simulink library "communications_lib"  (Simulink 8.1)
settings: Solver=ode45  StartTime=0.0  StopTime=10.0  RelTol=1e-3
values from neighbouring files (symbols this model uses):
  Ts = 100E-6    (= 0.0001)    [BANSHEE_init.m]
undefined symbols (not defined in the file or in its folder): DMS_slave_lib, DMSCommands
libraries: goose_lib x5, udp_powerfactor_lib x3, LoadProfiles_lib x1, NREL_UDP_lib x1, rtlab x1
settings Model: Creator=re25624  LastModifiedBy=pkoralew

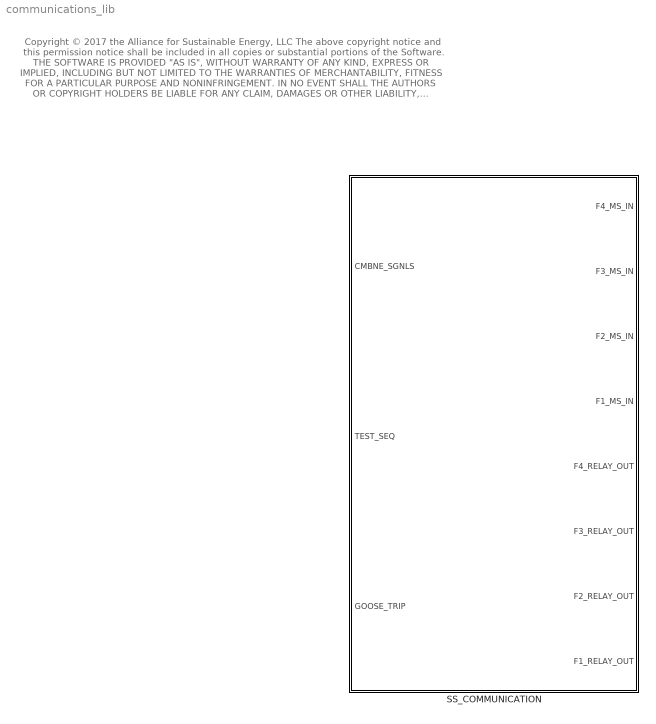
== system communications_lib ==
  note: Copyright © 2017 the Alliance for Sustainable Energy, LLC
      |
      | The above copyright notice and this permission notice shall be included in all copies or substantial portions of the Software.
      |
      | THE SOFTWARE IS PROVIDED "AS IS", WITHOUT WARRANTY OF ANY KIND, EXPRESS OR IMPLIED, INCLUDING
      | BUT NOT LIMITED TO THE WARRANTIES OF MERCHANTABILITY, FITNESS FOR A PARTICULAR PURPOSE AND
      | NONINFRINGEMENT. IN NO EVENT SHALL THE AUTHORS OR COPYRIGHT HOLDERS BE LIABLE FOR ANY CLAIM,
      |  DAMAGES OR OTHER LIABILITY, WHETHER IN AN ACTION OF CONTRACT, TORT OR OTHERWISE, ARISING FROM,
      | OUT OF OR IN CONNECTION WITH THE SOFTWARE OR THE USE OR OTHER DEALINGS IN THE SOFTWARE
  SS_COMMUNICATION : Subsystem

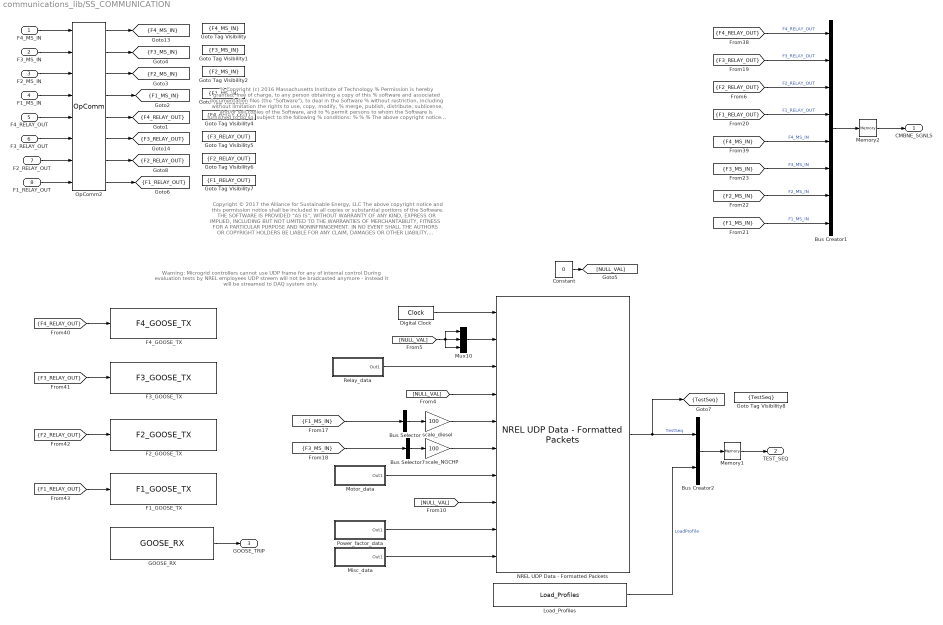
== system communications_lib/SS_COMMUNICATION ==
  note: Copyright © 2017 the Alliance for Sustainable Energy, LLC
      |
      | The above copyright notice and this permission notice shall be included in all copies or substantial portions of the Software.
      |
      | THE SOFTWARE IS PROVIDED "AS IS", WITHOUT WARRANTY OF ANY KIND, EXPRESS OR IMPLIED, INCLUDING
      | BUT NOT LIMITED TO THE WARRANTIES OF MERCHANTABILITY, FITNESS FOR A PARTICULAR PURPOSE AND
      | NONINFRINGEMENT. IN NO EVENT SHALL THE AUTHORS OR COPYRIGHT HOLDERS BE LIABLE FOR ANY CLAIM,
      |  DAMAGES OR OTHER LIABILITY, WHETHER IN AN ACTION OF CONTRACT, TORT OR OTHERWISE, ARISING FROM,
      | OUT OF OR IN CONNECTION WITH THE SOFTWARE OR THE USE OR OTHER DEALINGS IN THE SOFTWARE
  note: % Copyright (c) 2016 Massachusetts Institute of Technology
      | % Permission is hereby granted, free of charge, to any person obtaining a copy of this
      | % software and associated documentation files (the "Software"), to deal in the Software
      | % without restriction, including without limitation the rights to use, copy, modify,
      | % merge, publish, distribute, sublicense, and/or sell copies of the Software, and to
      | % permit persons to whom the Software is furnished to do so, subject to the following
      | % conditions:
      | %
      | %
      | % The above copyright notice and this permission notice shall be included in
      | % all copies or substantial portions of the Software.
      | %
      | % THE SOFTWARE IS PROVIDED "AS IS", WITHOUT WARRANTY OF ANY KIND, EXPRESS OR IMPLIED,
      | % INCLUDING BUT NOT LIMITED TO THE WARRANTIES OF MERCHANTABILITY, FITNESS FOR A
      | % PARTICULAR PURPOSE AND NONINFRINGEMENT. IN NO EVENT SHALL THE AUTHORS OR COPYRIGHT
      | % HOLDERS BE LIABLE FOR ANY CLAIM, DAMAGES OR OTHER LIABILITY, WHETHER IN AN ACTION
      | % OF CONTRACT, TORT OR OTHERWISE, ARISING FROM, OUT OF OR IN CONNECTION WITH THE
      | % SOFTWARE OR THE USE OR OTHER DEALINGS IN THE SOFTWARE.
      | %
      | %
      | %%
  note: Warning: Microgrid controllers cannot use UDP frame for any of internal control
      | During evaluation tests by NREL employees UDP streem will not be bradcasted anymore - instead it will
      | be streamed to DAQ system only.
  F4_MS_IN : Inport
  F3_MS_IN : Inport  Port=2
  F2_MS_IN : Inport  Port=3
  F1_MS_IN : Inport  Port=4
  F4_RELAY_OUT : Inport  Port=5
  F3_RELAY_OUT : Inport  Port=6
  F2_RELAY_OUT : Inport  Port=7
  F1_RELAY_OUT : Inport  Port=8
  Bus Creator1 : BusCreator  Inputs=8
  Bus Creator2 : BusCreator  Inputs=2
  Bus Selector : BusSelector  OutputSignals=DIESEL_DATA.gen.gal_per_hr,DIESEL_DATA.cb.relay_out.m.Vpu  OutputAsBus=on
  Bus Selector7 : BusSelector  OutputSignals=NG_CHP_DATA.cb.relay_out.m.Vpu,NG_CHP_DATA.CHPData.TempActual,NG_CHP_DATA.CHPData.Thermal data.Heat Recovered; MBtu/hr,NG_CHP_DATA.CHPData.Thermal data.Nm^3 per hour NG fuel usage,NG_CHP_DATA.CHPData.Thermal data.CO2 lbm/hr,NG_CHP_DATA.CHPData.HeatFromBoiler MBtu/hr,NG_CHP_DATA.CHPData.CHPHeatContribution MBtu/hr,NG_CHP_DATA.CHPData.Boiler_Nm^3/hr ,NG_CHP_DATA.CHPData.Boiler lbm/hr CO2  OutputAsBus=on
  Constant : Constant  Value=0
  Digital Clock : DigitalClock  SampleTime=Ts
  F1_GOOSE_TX : goose_lib/F1_GOOSE_TX
  F2_GOOSE_TX : goose_lib/F2_GOOSE_TX
  F3_GOOSE_TX : goose_lib/F3_GOOSE_TX
  F4_GOOSE_TX : goose_lib/F4_GOOSE_TX
  "GOOSE_RX " : goose_lib/GOOSE_RX 
  Goto Tag Visibility : GotoTagVisibility  GotoTag=F4_MS_IN
  Goto Tag Visibility1 : GotoTagVisibility  GotoTag=F3_MS_IN
  Goto Tag Visibility2 : GotoTagVisibility  GotoTag=F2_MS_IN
  Goto Tag Visibility3 : GotoTagVisibility  GotoTag=F1_MS_IN
  Goto Tag Visibility4 : GotoTagVisibility  GotoTag=F4_RELAY_OUT
  Goto Tag Visibility5 : GotoTagVisibility  GotoTag=F3_RELAY_OUT
  Goto Tag Visibility6 : GotoTagVisibility  GotoTag=F2_RELAY_OUT
  Goto Tag Visibility7 : GotoTagVisibility  GotoTag=F1_RELAY_OUT
  Goto Tag Visibility8 : GotoTagVisibility  GotoTag=TestSeq
  Load_Profiles : LoadProfiles_lib/Load_Profiles
  Memory1 : Memory
  Memory2 : Memory
  Misc_data : Subsystem
  Motor_data : Subsystem
  Mux10 : Mux  Inputs=3
  NREL UDP Data - Formatted Packets : NREL_UDP_lib/NREL UDP Data - Formatted Packets  ProfileID=2  NumOfWaveforms=[3, 1, 1]  NumOfRelays=[59, [1, 1, 1000, 100]]  NumOfBatteries=0  NumOfDieselGensets=[1, [100, 100]]  NumOfNGCHPGensets=[1, [100, 100, 100, 100, 100, 100, 100, 100, 100]]  NumOfMotors=2  NumOfPVs=0  NumOfPF=[3, 1000]  NumOfMiscellaneousDataScales=2  NumOfMiscellaneousDataSignalsScales=[[50, 1], [8, 1]]
  OpComm2 : rtlab/OpComm  nbport=8  groupe_acq=1  subsys_rate=0  st=0  Synchronization=on  Interpolation=on  Threshold=1.0  Missed_Data=off  Sim_Time=off  Samples=off  dynSigOut=off  from_console=0  warning_done=off  writeOpCommFile=off  Offset=off
  Power_factor_data : Subsystem
  Relay_data : Subsystem
  scale_NGCHP : Gain  Gain=100
  scale_diesel : Gain  Gain=100
  CMBNE_SGNLS : Outport
  TEST_SEQ : Outport  Port=2
  GOOSE_TRIP : Outport  Port=3
  tag scope: F1_MS_IN=scoped, F1_RELAY_OUT=scoped, F2_MS_IN=scoped, F2_RELAY_OUT=scoped, F3_MS_IN=scoped, F3_RELAY_OUT=scoped, F4_MS_IN=scoped, F4_RELAY_OUT=scoped, TestSeq=scoped
  wires:
  Bus Creator2/1 -> Memory1/1
  NREL UDP Data - Formatted Packets/1 -> Bus Creator2/1, [TestSeq]  "TestSeq"
  Motor_data/1(Out1) -> NREL UDP Data - Formatted Packets/7
  Misc_data/1(Out1) -> NREL UDP Data - Formatted Packets/10
  Relay_data/1(Out1) -> NREL UDP Data - Formatted Packets/3
  "GOOSE_RX "/1 -> GOOSE_TRIP/1
  [F1_RELAY_OUT] -> F1_GOOSE_TX/1
  [F2_RELAY_OUT] -> F2_GOOSE_TX/1
  [F3_RELAY_OUT] -> F3_GOOSE_TX/1
  [F4_RELAY_OUT] -> F4_GOOSE_TX/1
  [F4_MS_IN] -> Bus Creator1/5  "F4_MS_IN"
  [F4_RELAY_OUT] -> Bus Creator1/1  "F4_RELAY_OUT"
  OpComm2/8 -> [F1_RELAY_OUT]
  OpComm2/7 -> [F2_RELAY_OUT]
  OpComm2/6 -> [F3_RELAY_OUT]
  OpComm2/5 -> [F4_RELAY_OUT]
  OpComm2/4 -> [F1_MS_IN]
  OpComm2/3 -> [F2_MS_IN]
  OpComm2/2 -> [F3_MS_IN]
  OpComm2/1 -> [F4_MS_IN]
  F3_RELAY_OUT/1 -> OpComm2/6
  F4_RELAY_OUT/1 -> OpComm2/5
  F4_MS_IN/1 -> OpComm2/1
  Digital Clock/1 -> NREL UDP Data - Formatted Packets/1
  [F2_MS_IN] -> Bus Creator1/7  "F2_MS_IN"
  [F3_MS_IN] -> Bus Creator1/6  "F3_MS_IN"
  [F3_RELAY_OUT] -> Bus Creator1/2  "F3_RELAY_OUT"
  [F1_RELAY_OUT] -> Bus Creator1/4  "F1_RELAY_OUT"
  [F2_RELAY_OUT] -> Bus Creator1/3  "F2_RELAY_OUT"
  [F1_MS_IN] -> Bus Creator1/8  "F1_MS_IN"
  Bus Creator1/1 -> Memory2/1
  Memory2/1 -> CMBNE_SGNLS/1
  scale_NGCHP/1 -> NREL UDP Data - Formatted Packets/6
  Bus Selector7/1 -> scale_NGCHP/1
  scale_diesel/1 -> NREL UDP Data - Formatted Packets/5
  [F3_MS_IN] -> Bus Selector7/1
  Bus Selector/1 -> scale_diesel/1
  [F1_MS_IN] -> Bus Selector/1
  Power_factor_data/1(Out1) -> NREL UDP Data - Formatted Packets/9
  [NULL_VAL] -> NREL UDP Data - Formatted Packets/8
  [NULL_VAL] -> NREL UDP Data - Formatted Packets/4
  Constant/1 -> [NULL_VAL]
  Mux10/1 -> NREL UDP Data - Formatted Packets/2
  [NULL_VAL] -> Mux10/2, Mux10/1, Mux10/3
  F1_MS_IN/1 -> OpComm2/4
  F2_MS_IN/1 -> OpComm2/3
  F1_RELAY_OUT/1 -> OpComm2/8
  F2_RELAY_OUT/1 -> OpComm2/7
  Memory1/1 -> TEST_SEQ/1
  F3_MS_IN/1 -> OpComm2/2
  Load_Profiles/1 -> Bus Creator2/2  "LoadProfile"

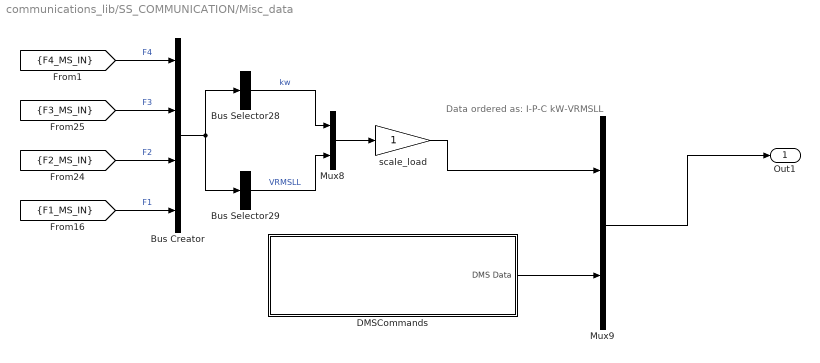
== system communications_lib/SS_COMMUNICATION/Misc_data ==
  note: Data ordered as:
      | I-P-C
      | kW-VRMSLL
  Bus Creator : BusCreator
  Bus Selector28 : BusSelector  OutputSignals=F1.LOAD_DATA.F1_I1.kw,F1.LOAD_DATA.F1_I2.kw,F2.LOAD_DATA.F2_I3.kw,F2.LOAD_DATA.F2_I4.kw,F2.LOAD_DATA.F2_I5.kw,F3.LOAD_DATA.F3_I6.kw,F4.LOAD_DATA.F4_I7.kw,F4.LOAD_DATA.F4_I8.kw,F1.LOAD_DATA.F1_P1.kw,F2.LOAD_DATA.F2_P2.kw,F2.LOAD_DATA.F2_P3.kw,F3.LOAD_DATA.F3_P4.kw,F2.LOAD_DATA.F2_P5.kw,F3.LOAD_DATA.F3_P6.kw,F4.LOAD_DATA.F4_P7.kw,F4.LOAD_DATA.F4_P8.kw,F1.LOAD_DATA.F1_C1.kw,F1.LOAD_DATA.F1_C2.kw,F2.LOAD_DATA.F2_C3.kw,F2.LOAD_DATA.F2_C4.kw,F3.LOAD_DATA.F3_C5.kw,F3.LOAD_DATA.F3_C6.kw,F4.LOAD_DATA.F4_C7.kw,F4.LOAD_DATA.F4_C8.kw,F4.LOAD_DATA.F4_C9.kw  OutputAsBus=on
  Bus Selector29 : BusSelector  OutputSignals=F1.LOAD_DATA.F1_I1.VRMSLL,F1.LOAD_DATA.F1_I2.VRMSLL,F2.LOAD_DATA.F2_I3.VRMSLL,F2.LOAD_DATA.F2_I4.VRMSLL,F2.LOAD_DATA.F2_I5.VRMSLL,F3.LOAD_DATA.F3_I6.VRMSLL,F4.LOAD_DATA.F4_I7.VRMSLL,F4.LOAD_DATA.F4_I8.VRMSLL,F1.LOAD_DATA.F1_P1.VRMSLL,F2.LOAD_DATA.F2_P2.VRMSLL,F2.LOAD_DATA.F2_P3.VRMSLL,F3.LOAD_DATA.F3_P4.VRMSLL,F2.LOAD_DATA.F2_P5.VRMSLL,F3.LOAD_DATA.F3_P6.VRMSLL,F4.LOAD_DATA.F4_P7.VRMSLL,F4.LOAD_DATA.F4_P8.VRMSLL,F1.LOAD_DATA.F1_C1.VRMSLL,F1.LOAD_DATA.F1_C2.VRMSLL,F2.LOAD_DATA.F2_C3.VRMSLL,F2.LOAD_DATA.F2_C4.VRMSLL,F3.LOAD_DATA.F3_C5.VRMSLL,F3.LOAD_DATA.F3_C6.VRMSLL,F4.LOAD_DATA.F4_C7.VRMSLL,F4.LOAD_DATA.F4_C8.VRMSLL,F4.LOAD_DATA.F4_C9.VRMSLL  OutputAsBus=on
  DMSCommands : Subsystem  AncestorBlock=DMS_slave_lib/DMSCommands
  Mux8 : Mux  Inputs=2
  Mux9 : Mux  Inputs=2
  scale_load : Gain
  Out1 : Outport
  wires:
  [F4_MS_IN] -> Bus Creator/1  "F4"
  Mux9/1 -> Out1/1
  DMSCommands/1(DMS Data) -> Mux9/2
  Mux8/1 -> scale_load/1
  Bus Selector29/1 -> Mux8/2  "VRMSLL"
  Bus Selector28/1 -> Mux8/1  "kw"
  Bus Creator/1 -> Bus Selector28/1, Bus Selector29/1
  [F1_MS_IN] -> Bus Creator/4  "F1"
  [F2_MS_IN] -> Bus Creator/3  "F2"
  [F3_MS_IN] -> Bus Creator/2  "F3"
  scale_load/1 -> Mux9/1

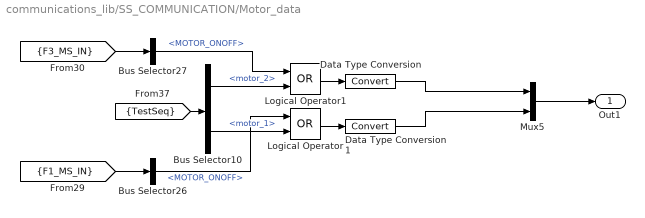
== system communications_lib/SS_COMMUNICATION/Motor_data ==
  Bus Selector10 : BusSelector  OutputSignals=motor_2,motor_1
  Bus Selector26 : BusSelector  OutputSignals=MOTOR_ONOFF
  Bus Selector27 : BusSelector  OutputSignals=MOTOR_ONOFF
  Data Type Conversion : DataTypeConversion
  Data Type Conversion1 : DataTypeConversion
  Logical Operator : Logic  Operator=OR  AllPortsSameDT=off  OutDataTypeStr=boolean
  Logical Operator1 : Logic  Operator=OR  AllPortsSameDT=off  OutDataTypeStr=boolean
  Mux5 : Mux  Inputs=2
  Out1 : Outport
  wires:
  Data Type Conversion/1 -> Mux5/1
  Data Type Conversion1/1 -> Mux5/2
  Logical Operator/1 -> Data Type Conversion1/1
  Logical Operator1/1 -> Data Type Conversion/1
  [F3_MS_IN] -> Bus Selector27/1
  [F1_MS_IN] -> Bus Selector26/1
  Bus Selector10/1 -> Logical Operator1/2  "<motor_2>"
  Bus Selector10/2 -> Logical Operator/2  "<motor_1>"
  [TestSeq] -> Bus Selector10/1
  Mux5/1 -> Out1/1
  Bus Selector26/1 -> Logical Operator/1  "<MOTOR_ONOFF>"
  Bus Selector27/1 -> Logical Operator1/1  "<MOTOR_ONOFF>"

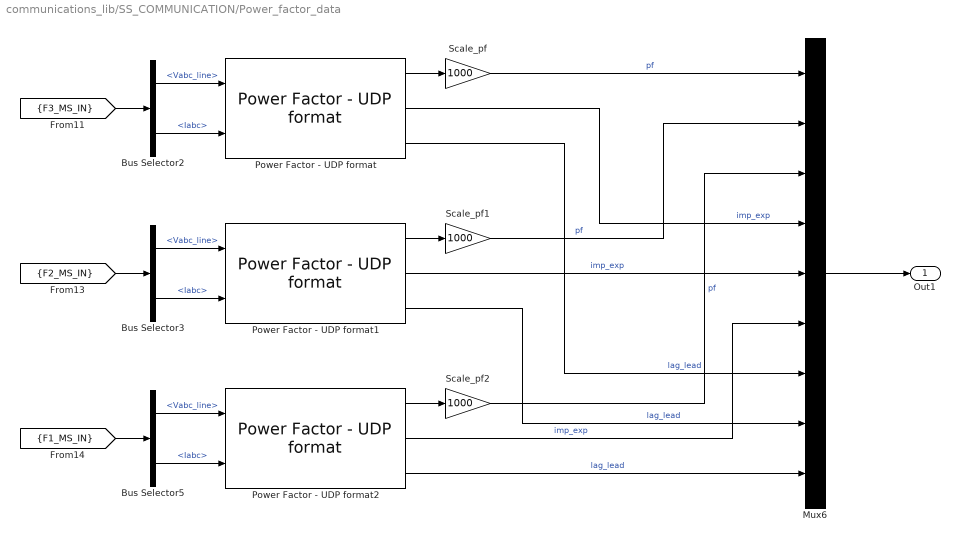
== system communications_lib/SS_COMMUNICATION/Power_factor_data ==
  Bus Selector2 : BusSelector  OutputSignals=CB_DATA.F3_PCC.Vabc_line,CB_DATA.F3_PCC.Iabc
  Bus Selector3 : BusSelector  OutputSignals=CB_DATA.F2_PCC.Vabc_line,CB_DATA.F2_PCC.Iabc
  Bus Selector5 : BusSelector  OutputSignals=CB_DATA.F1_PCC.Vabc_line,CB_DATA.F1_PCC.Iabc
  Mux6 : Mux  Inputs=9
  Power Factor - UDP format : udp_powerfactor_lib/Power Factor - UDP format
  Power Factor - UDP format1 : udp_powerfactor_lib/Power Factor - UDP format
  Power Factor - UDP format2 : udp_powerfactor_lib/Power Factor - UDP format
  Scale_pf : Gain  Gain=1000
  Scale_pf1 : Gain  Gain=1000
  Scale_pf2 : Gain  Gain=1000
  Out1 : Outport
  wires:
  Power Factor - UDP format2/3 -> Mux6/9  "lag_lead"
  Power Factor - UDP format1/3 -> Mux6/8  "lag_lead"
  Power Factor - UDP format/3 -> Mux6/7  "lag_lead"
  Power Factor - UDP format2/2 -> Mux6/6  "imp_exp"
  Power Factor - UDP format1/2 -> Mux6/5  "imp_exp"
  Power Factor - UDP format/2 -> Mux6/4  "imp_exp"
  Scale_pf2/1 -> Mux6/3  "pf"
  Scale_pf1/1 -> Mux6/2  "pf"
  Scale_pf/1 -> Mux6/1  "pf"
  Mux6/1 -> Out1/1
  Bus Selector5/2 -> Power Factor - UDP format2/2  "<Iabc>"
  Bus Selector5/1 -> Power Factor - UDP format2/1  "<Vabc_line>"
  Power Factor - UDP format2/1 -> Scale_pf2/1
  [F1_MS_IN] -> Bus Selector5/1
  Bus Selector3/2 -> Power Factor - UDP format1/2  "<Iabc>"
  Bus Selector3/1 -> Power Factor - UDP format1/1  "<Vabc_line>"
  Power Factor - UDP format1/1 -> Scale_pf1/1
  [F2_MS_IN] -> Bus Selector3/1
  Bus Selector2/2 -> Power Factor - UDP format/2  "<Iabc>"
  Bus Selector2/1 -> Power Factor - UDP format/1  "<Vabc_line>"
  Power Factor - UDP format/1 -> Scale_pf/1
  [F3_MS_IN] -> Bus Selector2/1

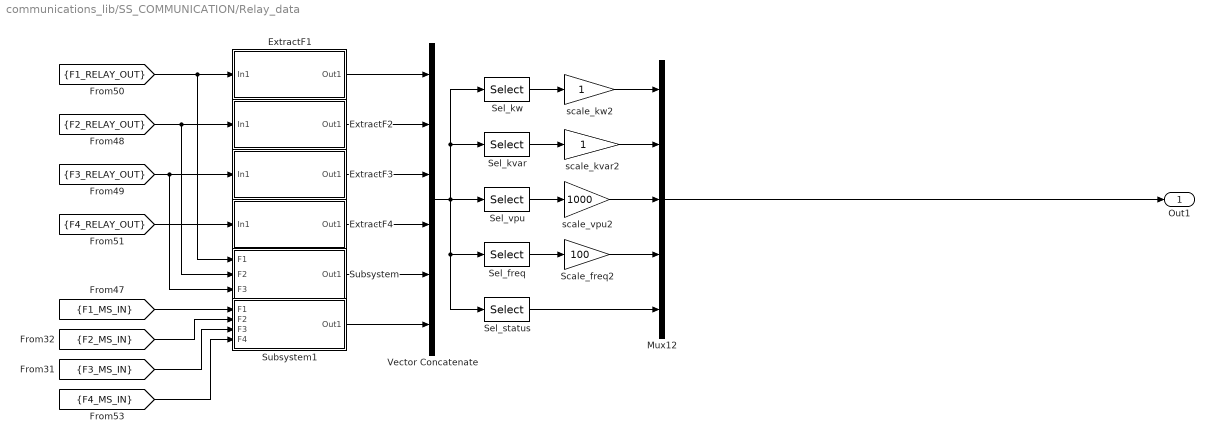
== system communications_lib/SS_COMMUNICATION/Relay_data ==
  ExtractF1 : Subsystem
      mask Display: disp('Generic F1 relays\nID = 01 .. 14')
  ExtractF2 : Subsystem
      mask Display: disp('Generic F2 relays\nID = 15 .. 33')
  ExtractF3 : Subsystem
      mask Display: disp('Generic F3 relays\nID = 34 .. 43')
  ExtractF4 : Subsystem
      mask Display: disp('Generic F4 relays\nID = 44 .. 49')
  Mux12 : Mux  Inputs=5
  Scale_freq2 : Gain  Gain=100
  Sel_freq : Selector  InputPortWidth=59*5  IndexOptions=Index vector (dialog)  Indices=[4:5:59*5]  OutputSizes=1
  Sel_kvar : Selector  InputPortWidth=59*5  IndexOptions=Index vector (dialog)  Indices=[2:5:59*5]  OutputSizes=1
  Sel_kw : Selector  InputPortWidth=59*5  IndexOptions=Index vector (dialog)  Indices=[1:5:59*5]  OutputSizes=1
  Sel_status : Selector  InputPortWidth=59*5  IndexOptions=Index vector (dialog)  Indices=[5:5:59*5]  OutputSizes=1
  Sel_vpu : Selector  InputPortWidth=59*5  IndexOptions=Index vector (dialog)  Indices=[3:5:59*5]  OutputSizes=1
  Subsystem : Subsystem
      mask Display: disp('Generic PCC relays\nID = 50 .. 52')
  Subsystem1 : Subsystem
      mask Display: disp('GEN1,ESS1,PV1\nGEN2,GEN3,ESS2,PV1\nID = 53 .. 59')
  Vector Concatenate : Concatenate  NumInputs=6
  scale_kvar2 : Gain
  scale_kw2 : Gain
  scale_vpu2 : Gain  Gain=1000
  Out1 : Outport
  wires:
  Vector Concatenate/1 -> Sel_kw/1, Sel_kvar/1, Sel_vpu/1, Sel_freq/1, Sel_status/1
  Sel_kvar/1 -> scale_kvar2/1
  Sel_vpu/1 -> scale_vpu2/1
  Sel_freq/1 -> Scale_freq2/1
  Sel_status/1 -> Mux12/5
  Sel_kw/1 -> scale_kw2/1
  scale_vpu2/1 -> Mux12/3
  Scale_freq2/1 -> Mux12/4
  scale_kvar2/1 -> Mux12/2
  scale_kw2/1 -> Mux12/1
  Mux12/1 -> Out1/1
  Subsystem1/1(Out1) -> Vector Concatenate/6
  [F1_MS_IN] -> Subsystem1/1(F1)
  [F2_MS_IN] -> Subsystem1/2(F2)
  [F3_MS_IN] -> Subsystem1/3(F3)
  [F4_MS_IN] -> Subsystem1/4(F4)
  Subsystem/1(Out1) -> Vector Concatenate/5
  ExtractF1/1(Out1) -> Vector Concatenate/1
  ExtractF2/1(Out1) -> Vector Concatenate/2
  ExtractF3/1(Out1) -> Vector Concatenate/3
  ExtractF4/1(Out1) -> Vector Concatenate/4
  [F4_RELAY_OUT] -> ExtractF4/1(In1)
  [F2_RELAY_OUT] -> ExtractF2/1(In1), Subsystem/2(F2)
  [F1_RELAY_OUT] -> ExtractF1/1(In1), Subsystem/1(F1)
  [F3_RELAY_OUT] -> ExtractF3/1(In1), Subsystem/3(F3)

== system communications_lib/SS_COMMUNICATION/Misc_data/DMSCommands ==
  note: Copyright (c) 2016 Massachusetts Institute of Technology
      | Permission is hereby granted, free of charge, to any person obtaining a copy of this software and associated documentation files (the "Software"), to deal
      | in the Software without restriction, including without limitation the rights to use, copy, modify, merge, publish, distribute, sublicense, and/or sell copies of the
      | Software, and to permit persons to whom the Software is furnished to do so, subject to the following conditions:
      |
      | THE SOFTWARE IS PROVIDED "AS IS", WITHOUT WARRANTY OF ANY KIND, EXPRESS OR IMPLIED, INCLUDING BUT NOT LIMITED TO THE
      | WARRANTIES OF MERCHANTABILITY, FITNESS FOR A PARTICULAR PURPOSE AND NONINFRINGEMENT. IN NO EVENT SHALL THE AUTHORS
      | OR COPYRIGHT HOLDERS BE LIABLE FOR ANY CLAIM, DAMAGES OR OTHER LIABILITY, WHETHER IN AN ACTION OF CONTRACT, TORT OR
      | OTHERWISE, ARISING FROM, OUT OF OR IN CONNECTION WITH THE SOFTWARE OR THE USE OR OTHER DEALINGS IN THE SOFTWARE
  Add : Sum
  Bus Creator : BusCreator  Inputs=8
  Constant : Constant  Value=zeros(1,12)
  Data Type Conversion : DataTypeConversion
  Demux : Demux  Outputs=11
  Gain : Gain  Gain=2^16
  Terminator : Terminator
  Terminator1 : Terminator
  DMS Data : Outport
  wires:
  Data Type Conversion/1 -> DMS Data/1
  Add/1 -> Bus Creator/1  "TimeStamp"
  Demux/1 -> Add/1
  Demux/2 -> Gain/1
  Gain/1 -> Add/2
  Constant/1 -> Demux/1
  Bus Creator/1 -> Data Type Conversion/1
  Demux/5 -> Bus Creator/2  "Disconnect"
  Demux/6 -> Bus Creator/3  "Limit Active"
  Demux/7 -> Bus Creator/4  "Limit Value"
  Demux/4 -> Terminator/1  "Fault2"
  Demux/3 -> Terminator1/1  "Fault1"
  Demux/8 -> Bus Creator/5  "PF Active"
  Demux/9 -> Bus Creator/6  "PF Value"
  Demux/10 -> Bus Creator/7  "VAR Active"
  Demux/11 -> Bus Creator/8  "VAR Value"

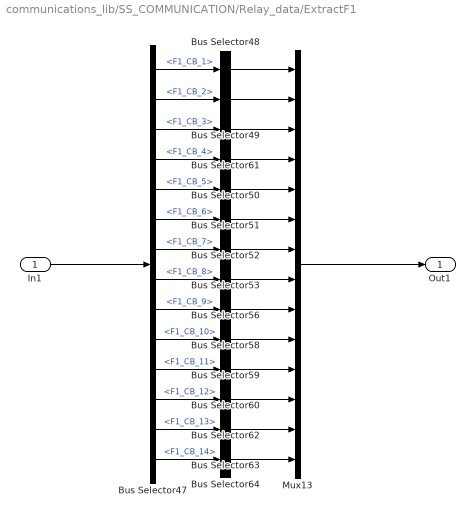
== system communications_lib/SS_COMMUNICATION/Relay_data/ExtractF1 ==
  In1 : Inport
  Bus Selector47 : BusSelector  OutputSignals=F1_CB_1,F1_CB_2,F1_CB_3,F1_CB_4,F1_CB_5,F1_CB_6,F1_CB_7,F1_CB_8,F1_CB_9,F1_CB_10,F1_CB_11,F1_CB_12,F1_CB_13,F1_CB_14
  Bus Selector{48..53,56,58..64} (14 alike) : BusSelector  OutputSignals=m.kw,m.kvar,m.Vpu,m.Hz,m.status  OutputAsBus=on
  Mux13 : Mux  Inputs=14
  Out1 : Outport
  wires:
  Bus Selector63/1 -> Mux13/13
  Bus Selector61/1 -> Mux13/3
  Bus Selector62/1 -> Mux13/12
  Bus Selector59/1 -> Mux13/10
  Bus Selector47/5 -> Bus Selector51/1  "<F1_CB_5>"
  Bus Selector47/10 -> Bus Selector59/1  "<F1_CB_10>"
  Bus Selector49/1 -> Mux13/2
  Bus Selector47/14 -> Bus Selector64/1  "<F1_CB_14>"
  Bus Selector47/2 -> Bus Selector49/1  "<F1_CB_2>"
  Bus Selector47/3 -> Bus Selector61/1  "<F1_CB_3>"
  Bus Selector47/9 -> Bus Selector58/1  "<F1_CB_9>"
  Bus Selector47/8 -> Bus Selector56/1  "<F1_CB_8>"
  Bus Selector47/12 -> Bus Selector62/1  "<F1_CB_12>"
  Bus Selector47/7 -> Bus Selector53/1  "<F1_CB_7>"
  Bus Selector64/1 -> Mux13/14
  Bus Selector47/6 -> Bus Selector52/1  "<F1_CB_6>"
  Bus Selector58/1 -> Mux13/9
  Bus Selector56/1 -> Mux13/8
  Bus Selector52/1 -> Mux13/6
  Bus Selector47/11 -> Bus Selector60/1  "<F1_CB_11>"
  Bus Selector60/1 -> Mux13/11
  Mux13/1 -> Out1/1
  In1/1 -> Bus Selector47/1
  Bus Selector50/1 -> Mux13/4
  Bus Selector47/1 -> Bus Selector48/1  "<F1_CB_1>"
  Bus Selector47/4 -> Bus Selector50/1  "<F1_CB_4>"
  Bus Selector53/1 -> Mux13/7
  Bus Selector48/1 -> Mux13/1
  Bus Selector51/1 -> Mux13/5
  Bus Selector47/13 -> Bus Selector63/1  "<F1_CB_13>"

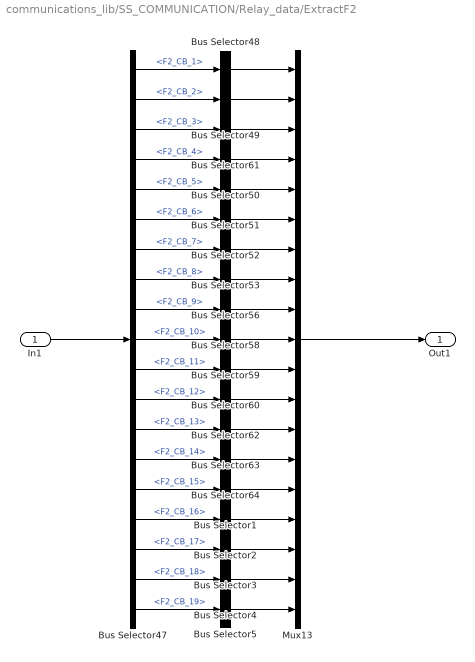
== system communications_lib/SS_COMMUNICATION/Relay_data/ExtractF2 ==
  In1 : Inport
  Bus Selector{1..5,48..53,56,58..64} (19 alike) : BusSelector  OutputSignals=m.kw,m.kvar,m.Vpu,m.Hz,m.status  OutputAsBus=on
  Bus Selector47 : BusSelector  OutputSignals=F2_CB_1,F2_CB_2,F2_CB_3,F2_CB_4,F2_CB_5,F2_CB_6,F2_CB_7,F2_CB_8,F2_CB_9,F2_CB_10,F2_CB_11,F2_CB_12,F2_CB_13,F2_CB_14,F2_CB_15,F2_CB_16,F2_CB_17,F2_CB_18,F2_CB_19
  Mux13 : Mux  Inputs=19
  Out1 : Outport
  wires:
  Bus Selector47/18 -> Bus Selector4/1  "<F2_CB_18>"
  Bus Selector2/1 -> Mux13/16
  Bus Selector47/16 -> Bus Selector2/1  "<F2_CB_16>"
  Bus Selector5/1 -> Mux13/19
  Bus Selector47/17 -> Bus Selector3/1  "<F2_CB_17>"
  Bus Selector47/19 -> Bus Selector5/1  "<F2_CB_19>"
  Bus Selector47/15 -> Bus Selector1/1  "<F2_CB_15>"
  Bus Selector1/1 -> Mux13/15
  Bus Selector3/1 -> Mux13/17
  Bus Selector4/1 -> Mux13/18
  Bus Selector47/13 -> Bus Selector63/1  "<F2_CB_13>"
  Bus Selector51/1 -> Mux13/5
  Bus Selector48/1 -> Mux13/1
  Bus Selector53/1 -> Mux13/7
  Bus Selector47/4 -> Bus Selector50/1  "<F2_CB_4>"
  Bus Selector47/1 -> Bus Selector48/1  "<F2_CB_1>"
  Bus Selector50/1 -> Mux13/4
  In1/1 -> Bus Selector47/1
  Mux13/1 -> Out1/1
  Bus Selector60/1 -> Mux13/11
  Bus Selector47/11 -> Bus Selector60/1  "<F2_CB_11>"
  Bus Selector52/1 -> Mux13/6
  Bus Selector56/1 -> Mux13/8
  Bus Selector58/1 -> Mux13/9
  Bus Selector47/6 -> Bus Selector52/1  "<F2_CB_6>"
  Bus Selector64/1 -> Mux13/14
  Bus Selector47/7 -> Bus Selector53/1  "<F2_CB_7>"
  Bus Selector47/12 -> Bus Selector62/1  "<F2_CB_12>"
  Bus Selector47/8 -> Bus Selector56/1  "<F2_CB_8>"
  Bus Selector47/9 -> Bus Selector58/1  "<F2_CB_9>"
  Bus Selector47/3 -> Bus Selector61/1  "<F2_CB_3>"
  Bus Selector47/2 -> Bus Selector49/1  "<F2_CB_2>"
  Bus Selector47/14 -> Bus Selector64/1  "<F2_CB_14>"
  Bus Selector49/1 -> Mux13/2
  Bus Selector47/10 -> Bus Selector59/1  "<F2_CB_10>"
  Bus Selector47/5 -> Bus Selector51/1  "<F2_CB_5>"
  Bus Selector59/1 -> Mux13/10
  Bus Selector62/1 -> Mux13/12
  Bus Selector61/1 -> Mux13/3
  Bus Selector63/1 -> Mux13/13

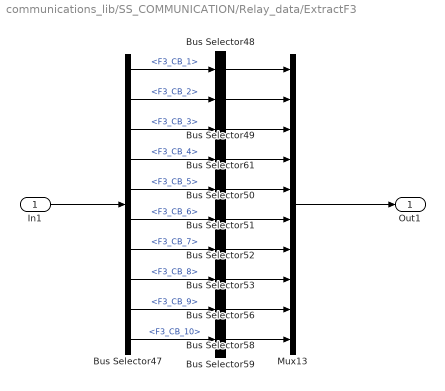
== system communications_lib/SS_COMMUNICATION/Relay_data/ExtractF3 ==
  In1 : Inport
  Bus Selector47 : BusSelector  OutputSignals=F3_CB_1,F3_CB_2,F3_CB_3,F3_CB_4,F3_CB_5,F3_CB_6,F3_CB_7,F3_CB_8,F3_CB_9,F3_CB_10
  Bus Selector{48..53,56,58..59,61} (10 alike) : BusSelector  OutputSignals=m.kw,m.kvar,m.Vpu,m.Hz,m.status  OutputAsBus=on
  Mux13 : Mux  Inputs=10
  Out1 : Outport
  wires:
  Bus Selector61/1 -> Mux13/3
  Bus Selector59/1 -> Mux13/10
  Bus Selector47/5 -> Bus Selector51/1  "<F3_CB_5>"
  Bus Selector47/10 -> Bus Selector59/1  "<F3_CB_10>"
  Bus Selector49/1 -> Mux13/2
  Bus Selector47/2 -> Bus Selector49/1  "<F3_CB_2>"
  Bus Selector47/3 -> Bus Selector61/1  "<F3_CB_3>"
  Bus Selector47/9 -> Bus Selector58/1  "<F3_CB_9>"
  Bus Selector47/8 -> Bus Selector56/1  "<F3_CB_8>"
  Bus Selector47/7 -> Bus Selector53/1  "<F3_CB_7>"
  Bus Selector47/6 -> Bus Selector52/1  "<F3_CB_6>"
  Bus Selector58/1 -> Mux13/9
  Bus Selector56/1 -> Mux13/8
  Bus Selector52/1 -> Mux13/6
  Mux13/1 -> Out1/1
  In1/1 -> Bus Selector47/1
  Bus Selector50/1 -> Mux13/4
  Bus Selector47/1 -> Bus Selector48/1  "<F3_CB_1>"
  Bus Selector47/4 -> Bus Selector50/1  "<F3_CB_4>"
  Bus Selector53/1 -> Mux13/7
  Bus Selector48/1 -> Mux13/1
  Bus Selector51/1 -> Mux13/5

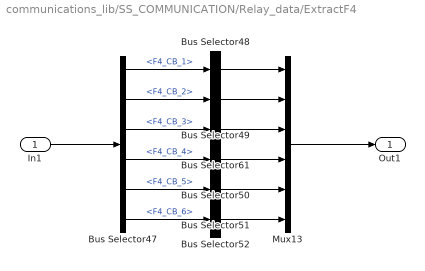
== system communications_lib/SS_COMMUNICATION/Relay_data/ExtractF4 ==
  In1 : Inport
  Bus Selector47 : BusSelector  OutputSignals=F4_CB_1,F4_CB_2,F4_CB_3,F4_CB_4,F4_CB_5,F4_CB_6
  Bus Selector{48..52,61} (6 alike) : BusSelector  OutputSignals=m.kw,m.kvar,m.Vpu,m.Hz,m.status  OutputAsBus=on
  Mux13 : Mux  Inputs=6
  Out1 : Outport
  wires:
  Bus Selector51/1 -> Mux13/5
  Bus Selector48/1 -> Mux13/1
  Bus Selector47/4 -> Bus Selector50/1  "<F4_CB_4>"
  Bus Selector47/1 -> Bus Selector48/1  "<F4_CB_1>"
  Bus Selector50/1 -> Mux13/4
  In1/1 -> Bus Selector47/1
  Mux13/1 -> Out1/1
  Bus Selector52/1 -> Mux13/6
  Bus Selector47/6 -> Bus Selector52/1  "<F4_CB_6>"
  Bus Selector47/3 -> Bus Selector61/1  "<F4_CB_3>"
  Bus Selector47/2 -> Bus Selector49/1  "<F4_CB_2>"
  Bus Selector49/1 -> Mux13/2
  Bus Selector47/5 -> Bus Selector51/1  "<F4_CB_5>"
  Bus Selector61/1 -> Mux13/3

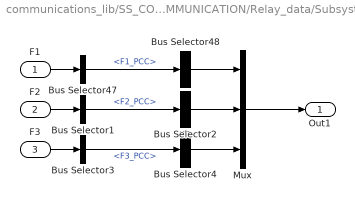
== system communications_lib/SS_COMMUNICATION/Relay_data/Subsystem ==
  F1 : Inport
  F2 : Inport  Port=2
  F3 : Inport  Port=3
  Bus Selector1 : BusSelector  OutputSignals=F2_PCC
  Bus Selector2 : BusSelector  OutputSignals=m.kw,m.kvar,m.Vpu,m.Hz,m.status  OutputAsBus=on
  Bus Selector3 : BusSelector  OutputSignals=F3_PCC
  Bus Selector4 : BusSelector  OutputSignals=m.kw,m.kvar,m.Vpu,m.Hz,m.status  OutputAsBus=on
  Bus Selector47 : BusSelector  OutputSignals=F1_PCC
  Bus Selector48 : BusSelector  OutputSignals=m.kw,m.kvar,m.Vpu,m.Hz,m.status  OutputAsBus=on
  Mux : Mux  Inputs=3
  Out1 : Outport
  wires:
  Mux/1 -> Out1/1
  Bus Selector4/1 -> Mux/3
  F3/1 -> Bus Selector3/1
  Bus Selector3/1 -> Bus Selector4/1  "<F3_PCC>"
  Bus Selector2/1 -> Mux/2
  F2/1 -> Bus Selector1/1
  Bus Selector1/1 -> Bus Selector2/1  "<F2_PCC>"
  Bus Selector48/1 -> Mux/1
  F1/1 -> Bus Selector47/1
  Bus Selector47/1 -> Bus Selector48/1  "<F1_PCC>"

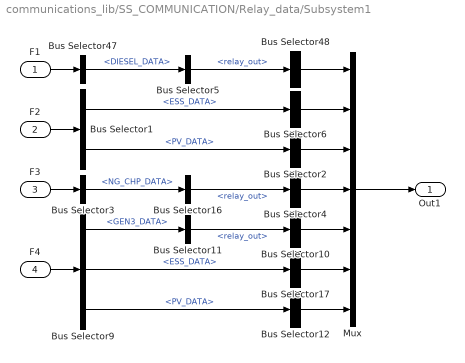
== system communications_lib/SS_COMMUNICATION/Relay_data/Subsystem1 ==
  F1 : Inport
  F2 : Inport  Port=2
  F3 : Inport  Port=3
  F4 : Inport  Port=4
  Bus Selector1 : BusSelector  OutputSignals=ESS_DATA,PV_DATA
  Bus Selector10 : BusSelector  OutputSignals=m.kw,m.kvar,m.Vpu,m.Hz,m.status  OutputAsBus=on
  Bus Selector11 : BusSelector  OutputSignals=cb.relay_out
  Bus Selector{2,6,12,17} (4 alike) : BusSelector  OutputSignals=CB_meas.relay_out.m.kw,CB_meas.relay_out.m.kvar,CB_meas.relay_out.m.Vpu,CB_meas.relay_out.m.Hz,CB_meas.cb_meas.Status  OutputAsBus=on
  Bus Selector16 : BusSelector  OutputSignals=cb.relay_out
  Bus Selector3 : BusSelector  OutputSignals=NG_CHP_DATA
  Bus Selector4 : BusSelector  OutputSignals=m.kw,m.kvar,m.Vpu,m.Hz,m.status  OutputAsBus=on
  Bus Selector47 : BusSelector  OutputSignals=DIESEL_DATA
  Bus Selector48 : BusSelector  OutputSignals=m.kw,m.kvar,m.Vpu,m.Hz,m.status  OutputAsBus=on
  Bus Selector5 : BusSelector  OutputSignals=cb.relay_out
  Bus Selector9 : BusSelector  OutputSignals=GEN3_DATA,ESS_DATA,PV_DATA
  Mux : Mux  Inputs=7
  Out1 : Outport
  wires:
  Bus Selector9/2 -> Bus Selector17/1  "<ESS_DATA>"
  Bus Selector16/1 -> Bus Selector4/1  "<relay_out>"
  Bus Selector12/1 -> Mux/7
  Bus Selector9/3 -> Bus Selector12/1  "<PV_DATA>"
  Bus Selector17/1 -> Mux/6
  Bus Selector10/1 -> Mux/5
  Bus Selector11/1 -> Bus Selector10/1  "<relay_out>"
  Bus Selector9/1 -> Bus Selector11/1  "<GEN3_DATA>"
  F4/1 -> Bus Selector9/1
  Bus Selector2/1 -> Mux/3
  Bus Selector1/2 -> Bus Selector2/1  "<PV_DATA>"
  Bus Selector5/1 -> Bus Selector48/1  "<relay_out>"
  Bus Selector47/1 -> Bus Selector5/1  "<DIESEL_DATA>"
  F1/1 -> Bus Selector47/1
  Bus Selector48/1 -> Mux/1
  Bus Selector1/1 -> Bus Selector6/1  "<ESS_DATA>"
  F2/1 -> Bus Selector1/1
  Bus Selector6/1 -> Mux/2
  Bus Selector3/1 -> Bus Selector16/1  "<NG_CHP_DATA>"
  F3/1 -> Bus Selector3/1
  Bus Selector4/1 -> Mux/4
  Mux/1 -> Out1/1
